simulink model "MultiCellInterface"  (Simulink 8.3)
settings: Solver=ode45  StartTime=0.0  StopTime=diga.daten.Programmdauer(end)  FixedStep=0.001  MaxStep=0.1  RelTol=1e-3
PostLoadFcn:
  | , if any(exist('dsrtsu_mdlpostloadfcn', 'file') == [2, 3, 6]), try dsrtsu_mdlpostloadfcn('Execute', bdroot); catch fprintf('Error in PostLoadFcn (dsrtsu_mdlpostloadfcn) for model "%s":\n %s\n', bdroot, lasterr); end, end,
  | ,try, asm_mdl_postloadfcn(bdroot, 'UpdateModel', 1300); catch, disp(lasterr); end,
libraries: balancing_strategies x1, MultiCellLibrary x1
settings Model: DSRTSU_INTERNAL_RTI_VER=450  DSRTSU_INTERNAL_RTI_TYPE=rti1006  DSRTSU_INTERNAL_RTIFPGA=40  Creator=fhu  LastModifiedBy=psa  BufferReuse=off
settings SolverCC: InitialStep=0.001
settings OptimizationCC: BlockReduction=off  OptimizeBlockIOStorage=off  BufferReuse=off  GlobalBufferReuse=off  ExpressionFolding=off  ExpressionDepthLimit=2147483647  LocalBlockOutputs=off
settings DebuggingCC: FcnCallInpInsideContextMsg=EnableAllAsWarning
settings HardwareCC: ProdIntDivRoundTo=Zero  ProdEndianess=LittleEndian  ProdHWDeviceType=Generic->Custom  TargetIntDivRoundTo=Zero  TargetEndianess=LittleEndian  TargetHWDeviceType=Generic->Custom
settings SFSimCC: SimUserLibraries=RTI\libISEAFrame.a
settings RTWCC: SystemTargetFile=rti1006.tlc  MakeCommand=make_rti  TemplateMakefile=rti1006.tmf  Description=dSPACE DS1006 Hardware Platform  ProcessScript=rti1006_make_rtw_hook
settings STFCustomTargetCC: ParMdlRefBuildCompliant=on  GeneratePreprocessorConditionals=Disable all  CPPClassGenCompliant=on  SystemTargetFile=rti1006.tlc
settings GRTTargetCC: CompOptLevelCompliant=off  ConcurrentExecutionCompliant=off  MatFileLogging=off  ExtModeMexFile=noextcomm
settings CustomProperty: DataType=RTWOptions_EnumType_C__Program Files (x86)_dSPACE RCPHIL 2014-B_MATLAB_RTI_RTI1006_TLC_rti1006_1InitialSimState  Value=RUN
settings EnumStrPairs: String=RUN

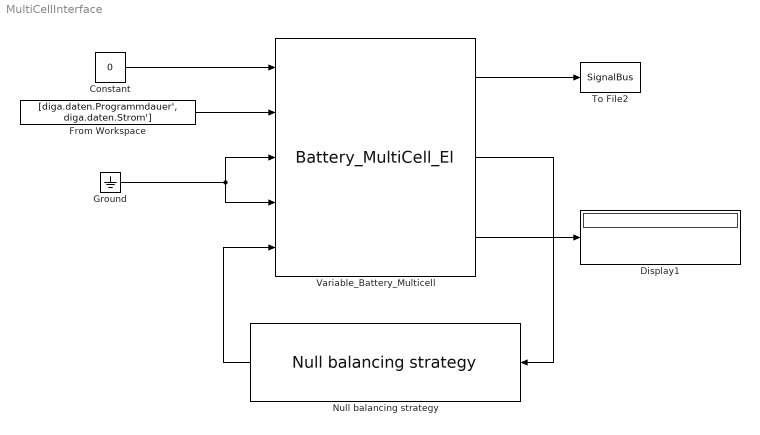
== system MultiCellInterface ==
  Constant : Constant  Value=0
  Display1 : Display
  From Workspace : FromWorkspace  VariableName=[diga.daten.Programmdauer', diga.daten.Strom']  SampleTime=0  Interpolate=off  OutputAfterFinalValue=Setting to zero
  Ground : Ground
  Null balancing strategy : balancing_strategies/Null balancing strategy
  To File2 : ToFile  Filename=SignalBus  MatrixName=SignalBus  SaveFormat=Timeseries
  Variable_Battery_Multicell : MultiCellLibrary/Battery_MultiCell_El  Tag=Battery_Multicell
  wires:
  Ground/1 -> Variable_Battery_Multicell/3, Variable_Battery_Multicell/4
  Variable_Battery_Multicell/3 -> Display1/1
  Null balancing strategy/1 -> Variable_Battery_Multicell/5
  Variable_Battery_Multicell/2 -> Null balancing strategy/1
  From Workspace/1 -> Variable_Battery_Multicell/2
  Variable_Battery_Multicell/1 -> To File2/1
  Constant/1 -> Variable_Battery_Multicell/1
